simulink model "p4"  (R2022b)
settings: Solver=VariableStepAuto  StartTime=0.0  StopTime=200  RelTol=1e-3
values from neighbouring files (symbols this model uses):
  Kp_PID = 1.2*Tp/(K*To)    (= 1.07071537472)    [pid_s1.m]
  Td_PID = 0.5*To    (= 0.625)    [pid_s1.m]
  Ti_PID = 2*To    (= 2.5)    [pid_s1.m]
libraries: fuzblock x1
settings Model: Creator=heloi  LastModifiedBy=heloi

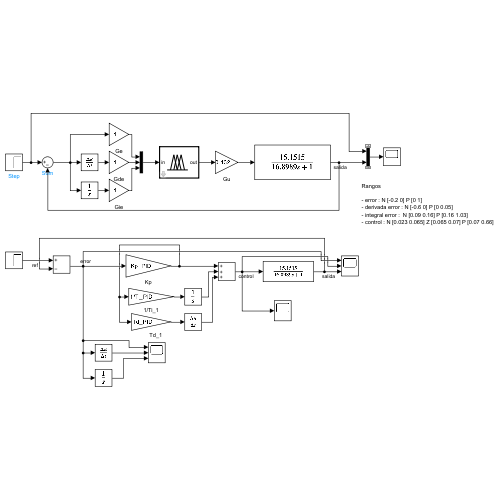
[thumbnail: Simulink's stored preview of the top-level diagram]
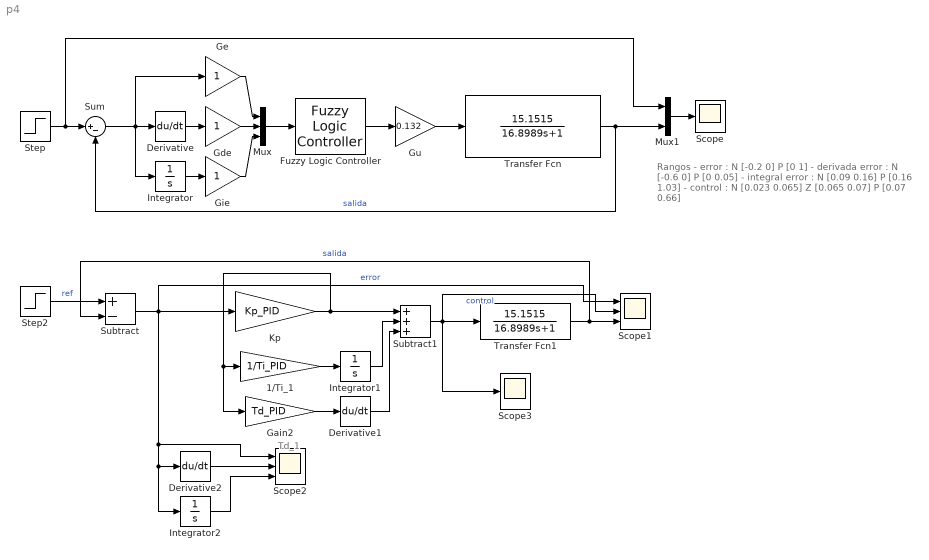
== system p4 ==
  note: Rangos
      |
      | - error : N [-0.2 0] P [0 1]
      | - derivada error : N [-0.6 0] P [0 0.05]
      | - integral error :  N [0.09 0.16] P [0.16 1.03]
      | - control : N [0.023 0.065] Z [0.065 0.07] P [0.07 0.66]
  note: Td_1
  1/Ti_1 : Gain  Gain=1/Ti_PID
  Derivative : Derivative
  Derivative1 : Derivative
  Derivative2 : Derivative
  Fuzzy Logic Controller : fuzblock/Fuzzy Logic  Controller  FIS='pid_fuzzy.fis'  OutputSampleNumber=101  DataType=double  FuzzifiedInputs=off  RuleFiringStrengths=off  RuleOutputs=off  AggregatedOutputs=off  SimulateUsing=Interpreted execution  OutOfRangeInputValueMessage=warning  NoRuleFiredMessage=warning  EmptyOutputFuzzySetMessage=warning
  Gain2 : Gain  Gain=Td_PID
  Gde : Gain
  Ge : Gain
  Gie : Gain
  Gu : Gain  Gain=0.132
  Integrator : Integrator
  Integrator1 : Integrator
  Integrator2 : Integrator
  Kp : Gain  Gain=Kp_PID
  Mux : Mux  Inputs=3
  Mux1 : Mux  Inputs=2
  Scope : Scope
  Scope1 : Scope  NumInputPorts=3
  Scope2 : Scope  NumInputPorts=3
  Scope3 : Scope
  Step : Step  SampleTime=0
  Step2 : Step  SampleTime=0
  Subtract : Sum  Inputs=+-
  Subtract1 : Sum  Inputs=+++
  Sum : Sum  Inputs=|+-
  Transfer Fcn : TransferFcn  Numerator=[15.1515]  Denominator=[16.8989 1]
  Transfer Fcn1 : TransferFcn  Numerator=15.1515  Denominator=[16.8989 1]
  wires:
  Step/1 -> Mux1/1, Sum/1
  Sum/1 -> Integrator/1, Ge/1, Derivative/1
  Derivative/1 -> Gde/1
  Transfer Fcn/1 -> Sum/2, Mux1/2  "salida"
  Mux1/1 -> Scope/1
  Mux/1 -> Fuzzy Logic Controller/1
  Fuzzy Logic Controller/1 -> Gu/1
  Derivative1/1 -> Subtract1/3
  Transfer Fcn1/1 -> Scope1/3, Subtract/2  "salida"
  Integrator1/1 -> Subtract1/2
  Gain2/1 -> Derivative1/1
  Subtract1/1 -> Scope1/2, Scope3/1, Transfer Fcn1/1  "control"
  1/Ti_1/1 -> Integrator1/1
  Kp/1 -> Subtract1/1, Gain2/1, 1/Ti_1/1
  Step2/1 -> Subtract/1  "ref"
  Subtract/1 -> Kp/1, Scope1/1, Scope2/1, Integrator2/1, Derivative2/1  "error"
  Derivative2/1 -> Scope2/2
  Integrator2/1 -> Scope2/3
  Gu/1 -> Transfer Fcn/1
  Ge/1 -> Mux/1
  Gde/1 -> Mux/2
  Integrator/1 -> Gie/1
  Gie/1 -> Mux/3
